simulink model "takeoff23b"  (R2025b)
settings: Solver=ode4  StartTime=0.0  StopTime=150  FixedStep=0.001  RelTol=1e-3
values from neighbouring files (symbols this model uses):
  a0 = 340.294    [basedata.m]    (also in basedata.mat; landing_init.m; landing_plan.mat; landingplan.mat)
  b_ref = 2.0    (= 2)    [basedata.m]    (also in basedata.mat; landing_init.m; landing_plan.mat; landingplan.mat)
  c_gear = [0.8e4, 1.4e4, 1.4e4]    [basedata.m]    (also in basedata.mat = [8000 14000 14000]; landing_init.m; landing_plan.mat = [8000 14000 14000]; landingplan.mat = [8000 14000 14000])
  c_lat = [1.4e4, 2.2e4, 2.2e4]    [basedata.m]    (also in basedata.mat = [14000 22000 22000]; landing_init.m; landing_plan.mat = [14000 22000 22000]; landingplan.mat = [14000 22000 22000])
  c_ref = 0.9    [basedata.m]    (also in basedata.mat; landing_init.m; landing_plan.mat; landingplan.mat)
  c_roll = [0.020, 0.018, 0.018]    [basedata.m]    (also in basedata.mat = [0.02 0.018 0.018]; landing_init.m; landing_plan.mat = [0.02 0.018 0.018]; landingplan.mat = [0.02 0.018 0.018])
  CD0 = 0.045    [basedata.m]    (also in basedata.mat; canshujisuan.m; landing_init.m; landing_plan.mat)
  CL0 = 0.083    [basedata.m]    (also in basedata.mat; landing_init.m; landing_plan.mat; landing_trajectory.m)
  CLa = 3.80    (= 3.8)    [basedata.m]    (also in basedata.mat; canshujisuan.m = 2.5; landing_init.m; landing_plan.mat)
  Clb = -0.08    [basedata.m]    (also in basedata.mat; landing_init.m; landing_plan.mat; landingplan.mat)
  Clda = -0.20    (= -0.2)    [basedata.m]    (also in basedata.mat; landing_init.m; landing_plan.mat; landingplan.mat)
  CLde = 0.28    [basedata.m]    (also in basedata.mat; landing_init.m; landing_plan.mat; landingplan.mat)
  Clp = -0.70    (= -0.7)    [basedata.m]    (also in basedata.mat; landing_init.m; landing_plan.mat; landingplan.mat)
  CLq = 4.50    (= 4.5)    [basedata.m]    (also in basedata.mat; canshujisuan.m = 3; landing_init.m; landing_plan.mat)
  Clr = 0.08    [basedata.m]    (also in basedata.mat; landing_init.m; landing_plan.mat; landingplan.mat)
  Cm0 = 0.060    (= 0.06)    [basedata.m]    (also in basedata.mat; landing_init.m; landing_plan.mat; landingplan.mat)
  Cma = -0.80    (= -0.8)    [basedata.m]    (also in basedata.mat; landing_init.m; landing_plan.mat; landingplan.mat)
  Cmde = -0.90    (= -0.9)    [basedata.m]    (also in basedata.mat; landing_init.m; landing_plan.mat; landingplan.mat)
  Cmq = -18.0    (= -18)    [basedata.m]    (also in basedata.mat; landing_init.m; landing_plan.mat; landingplan.mat)
  Cnb = 0.25    [basedata.m]    (also in basedata.mat; landing_init.m; landing_plan.mat; landingplan.mat)
  Cndr = -0.15    [basedata.m]    (also in basedata.mat; landing_init.m; landing_plan.mat; landingplan.mat)
  Cnp = -0.04    [basedata.m]    (also in basedata.mat; landing_init.m; landing_plan.mat; landingplan.mat)
  Cnr = -0.45    [basedata.m]    (also in basedata.mat; landing_init.m; landing_plan.mat; landingplan.mat)
  CSb = -0.70    (= -0.7)    [basedata.m]    (also in basedata.mat; landing_init.m; landing_plan.mat; landingplan.mat)
  CSdr = 0.18    [basedata.m]    (also in basedata.mat; landing_init.m; landing_plan.mat; landingplan.mat)
  CSr = 0.12    [basedata.m]    (also in basedata.mat; landing_init.m; landing_plan.mat; landingplan.mat)
  D = 0.5 * rho0 * V^2 * S_ref * CD_current    [canshujisuan.m]
  D0 = 1400    [basedata.m]    (also in basedata.mat; landing.m; landing_init.m; landing_plan.mat)
  da_max = 25    [basedata.m]    (also in basedata.mat; landing_init.m; landing_plan.mat; landingplan.mat)
  da_min = -da_max    (= -25)    [basedata.m]    (also in basedata.mat; landing_init.m; landing_plan.mat; landingplan.mat)
  de_max = 25    [basedata.m]    (also in basedata.mat; landing_init.m; landing_plan.mat; landingplan.mat)
  de_min = -de_max    (= -25)    [basedata.m]    (also in basedata.mat; landing_init.m; landing_plan.mat; landingplan.mat)
  DH = pi / 180    (= 0.0174532925199)    [basedata.m]    (also in basedata.mat; landing_init.m; landing_plan.mat; landingplan.mat)
  dr_max = 25    [basedata.m]    (also in basedata.mat; landing_init.m; landing_plan.mat; landingplan.mat)
  dr_min = -dr_max    (= -25)    [basedata.m]    (also in basedata.mat; landing_init.m; landing_plan.mat; landingplan.mat)
  g = 9.80665    [basedata.m]    (also in basedata.mat; canshujisuan.m; landing_init.m; landing_plan.mat)
  gamma1 = -0.125844364415    [basedata.mat]    (also in landing_trajectory.m = asin((T_idle - D_app) / (m*g)); landingplan.mat)
  gamma2 = -0.0261780104712    [basedata.mat]    (also in landing_trajectory.m; landingplan.mat)
  ground_z = 0.0    (= 0)    [basedata.m]    (also in basedata.mat; landing_init.m; landing_plan.mat; landingplan.mat)
  HD = 180 / pi    (= 57.2957795131)    [basedata.m]    (also in basedata.mat; landing_init.m; landing_plan.mat; landingplan.mat)
  I = [ Ixx, -Ixy, -Ixz ... (first row only)    [basedata.m]    (also in basedata.mat = [120  0  0; 0  480  0; 0  0  520]; landing_init.m; landing_plan.mat = [120  0  0; 0  480  0; 0  0  520]; landingplan.mat = [120  0  0; 0  480  0; 0  0  520])
  K = 0.12    [basedata.m]    (also in basedata.mat; canshujisuan.m = 0.08; landing_init.m; landing_plan.mat)
  K_alpha = 7.5375    [basedata.mat]    (also in control_design.m = (((wd_pitch^2)-a24))/(2*kesi_pitch*wd_pitch); control_design.mat; controller.m = 5; landingplan.mat)
  k_gear = [1.0e5, 3.0e5, 3.0e5]    [basedata.m]    (also in basedata.mat = [100000 300000 300000]; landing_init.m; landing_plan.mat = [100000 300000 300000]; landingplan.mat = [100000 300000 300000])
  Kn_pitch = -0.120095403309    [basedata.mat]    (also in control_design.m = -(2.2*g*(wd_pitch)^2)/(Tr*(((wd_pitch)^2)-a24)*V_control*a34; control_design.mat; controller.m = (2.2*wd^2*g)/(Tr*(wd^2-a24)*V_test*a34); landingplan.mat)
  Kw_pitch = -0.483749055178    [basedata.mat]    (also in control_design.m = -2*kesi_pitch*wd_pitch/a25; control_design.mat; controller.m = -(2*zeta*wd) / a25; landingplan.mat)
  m = 600.0    (= 600)    [basedata.m]    (also in basedata.mat; canshujisuan.m; landing_init.m; landing_plan.mat)
  mu_brake = [0.0, 0.55, 0.55]    [basedata.m]    (also in basedata.mat = [0 0.55 0.55]; landing_init.m; landing_plan.mat = [0 0.55 0.55]; landingplan.mat = [0 0.55 0.55])
  phi0 = 0.0    (= 0)    [landing.m]    (also in landing_init.m; landing_init.mat; landing_plan.mat; landingplan.mat)
  psi0 = 0.0    (= 0)    [landing.m]    (also in landing_init.m; landing_init.mat; landing_plan.mat; landingplan.mat)
  r_left_b = r_gear_b(:,2)    [basedata.m]    (also in basedata.mat = [-0.333333333333 -0.8 0.65]; landing_init.m; landing_plan.mat = [-0.333333333333 -0.8 0.65]; landingplan.mat = [-0.333333333333 -0.8 0.65])
  r_nose_b = r_gear_b(:,1)    [basedata.m]    (also in basedata.mat = [2 0 0.65]; landing_init.m; landing_plan.mat = [2 0 0.65]; landingplan.mat = [2 0 0.65])
  r_right_b = r_gear_b(:,3)    [basedata.m]    (also in basedata.mat = [-0.333333333333 0.8 0.65]; landing_init.m; landing_plan.mat = [-0.333333333333 0.8 0.65]; landingplan.mat = [-0.333333333333 0.8 0.65])
  rho0 = 1.225    [basedata.m]    (also in basedata.mat; canshujisuan.m; landing_init.m; landing_plan.mat)
  S_ref = 1.2    [basedata.m]    (also in basedata.mat; canshujisuan.m; landing_init.m; landing_plan.mat)
  theta0 = 0.0    (= 0)    [landing.m]    (also in landing_init.m; landing_init.mat = 0.0523598775598; landing_plan.mat = 0.0523560209424; landingplan.mat)
  u0_b = 128.0    (= 128)    [landing.m]    (also in landing_init.m; landing_init.mat = 100; landing_plan.mat; landingplan.mat)
  v0_b = 0.0    (= 0)    [landing.m]    (also in landing_init.m; landing_init.mat; landing_plan.mat; landingplan.mat)
  v_eps = 0.20    (= 0.2)    [basedata.m]    (also in basedata.mat; landing_init.m; landing_plan.mat; landingplan.mat)
  V_min = 3    [landing.m]    (also in landing_init.m; landing_plan.mat; landingplan.mat; plan.m = 1)
  w0_b = 0.0    (= 0)    [landing.m]    (also in landing_init.m; landing_init.mat; landing_plan.mat; landingplan.mat)
  wheel_radius = 0.18    [basedata.m]    (also in basedata.mat; landing_init.m; landing_plan.mat; landingplan.mat)
  WOW_on = 0.000    (= 0)    [basedata.m]    (also in basedata.mat; landing_init.m; landing_plan.mat; landingplan.mat)
  Xg0 = -12000.0    (= -12000)    [landing.m]    (also in landing_init.m; landing_init.mat = -8000; landing_plan.mat; landingplan.mat)
  Yg0 = 0.0    (= 0)    [landing.m]    (also in landing_init.m; landing_init.mat; landing_plan.mat; landingplan.mat)
  Zg0 = ground_z - wheel_radius - r_gear_b(3,1) + static_deflection    [basedata.m]    (also in basedata.mat = -0.8215943; landing.m = -1000; landing_init.m = -1000; landing_init.mat = -350)
undefined symbols (not defined in the file or in its folder): I_xz, I_yz, Ix_Iy, Iy_Iz, Iz_Ix
libraries: simulink x58, matrix_library x19
(part 2 of 4)

== system takeoff23b/Guidance/4_拉平制导 ==
  h_ALG : Inport
  h_dot : Inport  Port=2
  e_Z : Inport  Port=3
  e_psi : Inport  Port=4
  Enable : EnablePort
  Add : Sum  Inputs=+-
  Add1 : Sum  Inputs=+-
  Add2 : Sum
  Add3 : Sum  Inputs=+-
  Bus Creator : BusCreator  Inputs=10
  Constant : Constant  Value=-0.5
  Constant1 : Constant
  Constant2 : Constant  Value=0
  Constant3 : Constant  Value=0
  Gain : Gain  Gain=-1/2
  Gain1 : Gain  Gain=0.2
  Gain2 : Gain  Gain=-1
  Gain3 : Gain  Gain=-1
  Gain4 : Gain  Gain=0.02
  Gain5 : Gain  Gain=0.5
  H_cmd : Constant  Value=0
  Saturation : Saturate  UpperLimit=1.5  LowerLimit=0
  Saturation1 : Saturate  UpperLimit=0.17  LowerLimit=-0.17
  V_cmd : Constant  Value=200
  brake_cmd : Constant  Value=0
  gamma : Constant  Value=0
  theta_cmd : Constant  Value=0
  throttle_cmd : Constant  Value=0
  cmd_Bus : Outport
  wires:
  brake_cmd/1 -> Bus Creator/8  "brake_cmd"
  Saturation1/1 -> Bus Creator/4  "psi_cmd"
  V_cmd/1 -> Bus Creator/6  "V_cmd"
  throttle_cmd/1 -> Bus Creator/7  "throttle_cmd"
  Saturation/1 -> Bus Creator/1  "nz_cmd"
  theta_cmd/1 -> Bus Creator/5  "theta_cmd"
  Constant3/1 -> Bus Creator/2  "ny_cmd"
  Bus Creator/1 -> cmd_Bus/1
  Constant2/1 -> Bus Creator/3  "phi_cmd"
  h_ALG/1 -> Add/1
  Constant/1 -> Add/2
  Add/1 -> Gain/1
  h_dot/1 -> Add1/1
  Gain/1 -> Add1/2
  Gain1/1 -> Add2/1
  Add1/1 -> Gain1/1
  Constant1/1 -> Add2/2
  Add2/1 -> Saturation/1
  e_Z/1 -> Gain2/1
  e_psi/1 -> Gain3/1
  Gain2/1 -> Gain4/1
  Gain3/1 -> Gain5/1
  Gain4/1 -> Add3/1
  Gain5/1 -> Add3/2
  Add3/1 -> Saturation1/1
  H_cmd/1 -> Bus Creator/10  "H_cmd"
  gamma/1 -> Bus Creator/9  "gamma"

== system takeoff23b/controller1/1_Pitch_Ctrl ==
  Flight_Phase : Inport
  nz_cmd : Inport  Port=2
  theta_cmd : Inport  Port=3
  nz : Inport  Port=4
  theta : Inport  Port=5
  q : Inport  Port=6
  H_cmd : Inport  Port=7
  gamma : Inport  Port=8
  234俯仰角控制 : Subsystem
  5_着陆俯仰控制 : Subsystem
  5三回路控制 : Subsystem
  Clock_blend : Clock
  Compare To Constant1 : simulink/Logic and Bit Operations/Compare To Constant  relop=>=  const=6  OutDataTypeStr=boolean
  Compare To Constant2 : simulink/Logic and Bit Operations/Compare To Constant  relop=>=  const=5  OutDataTypeStr=boolean
  Compare To Constant3 : simulink/Logic and Bit Operations/Compare To Constant  relop=<=  const=9  OutDataTypeStr=boolean
  Compare To Constant4 : simulink/Logic and Bit Operations/Compare To Constant  relop=<=  const=7  OutDataTypeStr=boolean
  Gain3 : Gain  Gain=180/pi
  Logical Operator1 : Logic  AllPortsSameDT=off  OutDataTypeStr=boolean
  Logical Operator2 : Logic  Operator=NOT  AllPortsSameDT=off  OutDataTypeStr=boolean
  Logical Operator3 : Logic  AllPortsSameDT=off  OutDataTypeStr=boolean
  Pitch45Blend : MATLAB Function  TreatAsAtomicUnit=on  SystemSampleTime=0.001
  Saturation : Saturate  UpperLimit=25  LowerLimit=-25
  Scope1 : Scope
      settings: ActiveDisplayYMinimum=-0.125  ActiveDisplayYMaximum=1.125
  Scope2 : Scope
      settings: ActiveDisplayYMinimum=-3.5044630346224475  ActiveDisplayYMaximum=0.72101097537351044  DataLoggingVariableName=ScopeData30
  Switch : Switch  Criteria=u2 > Threshold  SaturateOnIntegerOverflow=off  InputSameDT=off
  T_blend : Constant  Value=5
  de_cmd : Outport
  wires:
  Pitch45Blend/1(de_cmd_rad) -> Gain3/1
  Compare To Constant3/1 -> Logical Operator1/1
  Compare To Constant2/1 -> Logical Operator1/2
  Logical Operator1/1 -> Logical Operator2/1
  Flight_Phase/1 -> Compare To Constant3/1, Pitch45Blend/1(phase), Compare To Constant4/1, Compare To Constant1/1, Compare To Constant2/1
  Clock_blend/1 -> Pitch45Blend/4(t)
  Pitch45Blend/2(lambda) -> Scope1/1
  T_blend/1 -> Pitch45Blend/5(T_blend)
  Gain3/1 -> Saturation/1
  theta_cmd/1 -> 234俯仰角控制/1(theta_cmd)
  theta/1 -> 234俯仰角控制/2(theta)
  nz_cmd/1 -> 5三回路控制/1(nz_cmd)
  nz/1 -> 5三回路控制/2(nz)
  q/1 -> 234俯仰角控制/3(q), 5三回路控制/3(q)
  Logical Operator2/1 -> 5三回路控制/4(复位)
  234俯仰角控制/1(de_theta_rad) -> Pitch45Blend/2(de_theta_rad)
  5三回路控制/1(de_nz_rad) -> Switch/1, Pitch45Blend/3(de_ny_rad)
  Compare To Constant1/1 -> Logical Operator3/2
  Compare To Constant4/1 -> Logical Operator3/1
  Logical Operator3/1 -> Switch/2
  Switch/1 -> Scope2/1, de_cmd/1
  5_着陆俯仰控制/1(de) -> Switch/3
  [Vg] -> 5_着陆俯仰控制/1(Vg)
  H_cmd/1 -> 5_着陆俯仰控制/3(h_com)
  gamma/1 -> 5_着陆俯仰控制/2(gamma)

== system takeoff23b/controller1/2_Yaw_Ctrl ==
  Flight_Phase : Inport
  psi_cmd : Inport  Port=2
  Y : Inport  Port=3
  psi : Inport  Port=4
  r : Inport  Port=5
  2345上升段控制 : Subsystem
  Compare To Constant : simulink/Logic and Bit Operations/Compare To Constant  relop=>=  const=1  OutDataTypeStr=boolean
  Compare To Constant1 : simulink/Logic and Bit Operations/Compare To Constant  relop=<=  const=8  OutDataTypeStr=boolean
  Compare To Constant2 : simulink/Logic and Bit Operations/Compare To Constant  relop===  const=1  OutDataTypeStr=boolean
  Compare To Constant3 : simulink/Logic and Bit Operations/Compare To Constant  relop===  const=10  OutDataTypeStr=boolean
  Compare To Constant4 : simulink/Logic and Bit Operations/Compare To Constant  relop===  const=11  OutDataTypeStr=boolean
  Constant : Constant  Value=0
  Constant1 : Constant  Value=0
  Gain : Gain  Gain=180/pi
  Gain1 : Gain  Gain=180/pi
  Logical Operator : Logic  AllPortsSameDT=off  OutDataTypeStr=boolean
  Logical Operator1 : Logic  Operator=OR  Inputs=3  AllPortsSameDT=off  OutDataTypeStr=boolean
  Saturation : Saturate  UpperLimit=25  LowerLimit=-25
  Saturation1 : Saturate  UpperLimit=25  LowerLimit=-25
  Scope : Scope
      settings: ActiveDisplayYMinimum=-0.036  ActiveDisplayYMaximum=0.004
  Switch : Switch  Criteria=u2 > Threshold  SaturateOnIntegerOverflow=off  InputSameDT=off
  Switch1 : Switch  Criteria=u2 > Threshold  SaturateOnIntegerOverflow=off  InputSameDT=off
  dr_cmd : Outport
  delta_s_cmd : Outport  Port=2
  wires:
  Gain/1 -> Saturation/1
  Saturation/1 -> dr_cmd/1
  Saturation1/1 -> delta_s_cmd/1
  Gain1/1 -> Saturation1/1
  Compare To Constant/1 -> Logical Operator/1
  Compare To Constant1/1 -> Logical Operator/2
  Logical Operator/1 -> Switch/2
  Compare To Constant3/1 -> Logical Operator1/2
  Compare To Constant2/1 -> Logical Operator1/1
  Compare To Constant4/1 -> Logical Operator1/3
  Logical Operator1/1 -> Switch1/2
  Constant/1 -> Switch1/3
  Flight_Phase/1 -> Compare To Constant/1, Compare To Constant1/1, Compare To Constant2/1, Compare To Constant3/1, Compare To Constant4/1
  Constant1/1 -> Switch/3  "阶段9"
  Switch1/1 -> Gain1/1
  Switch/1 -> Gain/1
  2345上升段控制/1(dr_cmd) -> Switch/1
  psi_cmd/1 -> Switch1/1
  Y/1 -> 2345上升段控制/1(Y)
  psi/1 -> Scope/1, 2345上升段控制/2(psi)
  r/1 -> 2345上升段控制/3(r)
  [Vwind_ground] -> 2345上升段控制/4(Vwind_ground)
  [Va_safe] -> 2345上升段控制/5(Va_safe)

== system takeoff23b/controller1/3_Roll_Ctrl ==
  phi_cmd : Inport
  phi : Inport  Port=2
  p : Inport  Port=3
  Gain : Gain  Gain=180/pi
  Gain1 : Gain
  Gain2 : Gain  Gain=5
  Gain3 : Gain  Gain=0.1
  Gain4 : Gain  Gain=-1
  Integrator : Integrator
  Saturation : Saturate  UpperLimit=25  LowerLimit=-25
  Saturation1 : Saturate  UpperLimit=0.52  LowerLimit=-0.52
  Sum : Sum  Inputs=|+-
  Sum1 : Sum  Inputs=|++
  Sum2 : Sum  Inputs=|+-
  da_cmd : Outport
  wires:
  Gain/1 -> Saturation/1
  Saturation/1 -> Gain4/1
  phi_cmd/1 -> Sum/1
  phi/1 -> Sum/2
  Sum/1 -> Saturation1/1
  Gain3/1 -> Integrator/1
  Integrator/1 -> Sum1/2
  Gain2/1 -> Sum1/1
  Sum1/1 -> Sum2/1
  p/1 -> Sum2/2
  Sum2/1 -> Gain1/1
  Saturation1/1 -> Gain2/1, Gain3/1
  Gain1/1 -> Gain/1
  Gain4/1 -> da_cmd/1

== system takeoff23b/controller1/4_Power&V_Ctrl ==
  Flight_Phase : Inport
  V_cmd : Inport  Port=2
  throttle_cmd : Inport  Port=3
  V : Inport  Port=4
  brake_cmd : Inport  Port=5
  Clock_blend : Clock
  Constant : Constant  Value=3
  Delay : Delay  DelayLength=1
  Gain : Gain  Gain=0.1
  Gain1 : Gain  Gain=0.08
  MATLAB Function : MATLAB Function  TreatAsAtomicUnit=on
  MATLAB Function1 : MATLAB Function  TreatAsAtomicUnit=on
  Max : MinMax  Function=max  Inputs=2
  Saturation : Saturate  UpperLimit=0.55  LowerLimit=-0.45
  Saturation1 : Saturate  UpperLimit=1  LowerLimit=0
  Saturation2 : Saturate  UpperLimit=1  LowerLimit=0
  Scope : Scope
      settings: DataLoggingVariableName=ScopeData3
  Sum1 : Sum  Inputs=|+-
  Sum2 : Sum  Inputs=|++
  Sum3 : Sum  Inputs=|+-
  平衡油门 : Constant  Value=0.45
  最小爬升油门保护 : Constant  Value=0.3
  throttle : Outport
  u_brake_cmd : Outport  Port=2
  wires:
  Saturation1/1 -> u_brake_cmd/1
  V/1 -> Sum3/2
  V_cmd/1 -> Sum3/1
  brake_cmd/1 -> Saturation1/1
  Sum3/1 -> Gain/1
  Gain/1 -> Sum1/1
  Sum1/1 -> Saturation/1
  平衡油门/1 -> Sum2/2
  [vg_xyz] -> MATLAB Function/1(Vel_g)
  [a_xyz] -> MATLAB Function/2(axyz)
  MATLAB Function/1(dv_err) -> Delay/1
  Gain1/1 -> Sum1/2
  Saturation/1 -> Sum2/1
  Sum2/1 -> Max/1
  Clock_blend/1 -> MATLAB Function1/4(t)
  throttle_cmd/1 -> MATLAB Function1/2(throttle_direct)
  Max/1 -> MATLAB Function1/3(throttle_speed)
  Flight_Phase/1 -> MATLAB Function1/1(phase)
  Constant/1 -> MATLAB Function1/5(T_blend)
  MATLAB Function1/1(throttle_out) -> Saturation2/1
  MATLAB Function1/2(lambda) -> Scope/1
  Delay/1 -> Gain1/1
  Saturation2/1 -> throttle/1

== system takeoff23b/controller1/刹车 ==
  u_brake_cmd : Inport
  Gain : Gain  Gain=1/0.1
  Integrator : Integrator  LimitOutput=on  UpperSaturationLimit=1  LowerSaturationLimit=0
  Sum : Sum  Inputs=|+-
  限制舵面角速度 : Saturate  UpperLimit=5  LowerLimit=-5
  u_brake : Outport
  wires:
  u_brake_cmd/1 -> Sum/1
  Sum/1 -> Gain/1
  Gain/1 -> 限制舵面角速度/1
  限制舵面角速度/1 -> Integrator/1
  Integrator/1 -> Sum/2, u_brake/1

== system takeoff23b/controller1/前轮 ==
  delta_s_cmd : Inport
  Gain : Gain  Gain=1/0.08
  Integrator : Integrator  LimitOutput=on  UpperSaturationLimit=25  LowerSaturationLimit=-25
  Sum : Sum  Inputs=|+-
  限制偏转速度 : Saturate  UpperLimit=120  LowerLimit=-120
  delta_s : Outport
  wires:
  delta_s_cmd/1 -> Sum/1
  Sum/1 -> Gain/1
  Gain/1 -> 限制偏转速度/1
  限制偏转速度/1 -> Integrator/1
  Integrator/1 -> Sum/2, delta_s/1

== system takeoff23b/controller1/副翼 ==
  da_cmd : Inport
  Gain : Gain  Gain=1/0.05
  Integrator : Integrator  LimitOutput=on  UpperSaturationLimit=25  LowerSaturationLimit=-25
  Sum : Sum  Inputs=|+-
  限制舵面角速度 : Saturate  UpperLimit=120  LowerLimit=-120
  da : Outport
  wires:
  da_cmd/1 -> Sum/1
  Sum/1 -> Gain/1
  Gain/1 -> 限制舵面角速度/1
  限制舵面角速度/1 -> Integrator/1
  Integrator/1 -> Sum/2, da/1

== system takeoff23b/controller1/升降舵 ==
  de_cmd : Inport
  Gain : Gain  Gain=1/0.08
  Integrator : Integrator  LimitOutput=on  UpperSaturationLimit=25  LowerSaturationLimit=-25
  Sum : Sum  Inputs=|+-
  限制舵面角速度 : Saturate  UpperLimit=50  LowerLimit=-50
  de : Outport
  wires:
  de_cmd/1 -> Sum/1
  Sum/1 -> Gain/1
  Gain/1 -> 限制舵面角速度/1
  限制舵面角速度/1 -> Integrator/1
  Integrator/1 -> Sum/2, de/1

== system takeoff23b/controller1/方向舵 ==
  dr_cmd : Inport
  Gain : Gain  Gain=1/0.05
  Integrator : Integrator  LimitOutput=on  UpperSaturationLimit=25  LowerSaturationLimit=-25
  Sum : Sum  Inputs=|+-
  限制舵面角速度 : Saturate  UpperLimit=100  LowerLimit=-100
  dr : Outport
  wires:
  Integrator/1 -> dr/1, Sum/2
  限制舵面角速度/1 -> Integrator/1
  Gain/1 -> 限制舵面角速度/1
  Sum/1 -> Gain/1
  dr_cmd/1 -> Sum/1

== system takeoff23b/controller1/油门 ==
  throttle : Inport
  Constant : Constant  Value=3000
  Gain : Gain  Gain=1/0.5
  Integrator : Integrator  LimitOutput=on  UpperSaturationLimit=1  LowerSaturationLimit=0
  Product : Product
  Saturation : Saturate  UpperLimit=3  LowerLimit=-3
  Sum : Sum  Inputs=|+-
  thrust : Outport
  wires:
  Integrator/1 -> Product/2, Sum/2
  Saturation/1 -> Integrator/1
  Gain/1 -> Saturation/1
  Sum/1 -> Gain/1
  throttle/1 -> Sum/1
  Product/1 -> thrust/1
  Constant/1 -> Product/1

== system takeoff23b/6DOF-MODEL/AERO-PARAMETER/atmosphere ==
  Constant : Constant  Value=0
  Constant1 : Constant  Value=rho0
  Constant2 : Constant  Value=a0
  Constant3 : Constant  Value=0.5
  Constant4 : Constant  Value=0
  Constant5 : Constant  Value=0
  Display : Display
  MATLAB Function : MATLAB Function  TreatAsAtomicUnit=on
  Matrix Multiply : Product  Multiplication=Matrix(*)
  Mux : Mux  Inputs=3
  Product : Product  Inputs=3
  Reshape : Reshape  OutputDimensionality=Column vector (2-D)
  Square : Math  Operator=square
  tag scope: Vwind_body=global, Vwind_ground=global, a_sound=global, qc=global, rho=global
  wires:
  Constant1/1 -> [rho]
  Constant2/1 -> [a_sound]
  Constant3/1 -> Product/1
  [rho] -> Product/2
  Product/1 -> Display/1, [qc]
  Square/1 -> Product/3
  [Vg] -> Square/1
  Constant5/1 -> Mux/2
  Constant4/1 -> Mux/1
  Constant/1 -> Mux/3
  Mux/1 -> Reshape/1
  Reshape/1 -> [Vwind_ground]
  [Vwind_ground] -> Matrix Multiply/2
  [theta_eular] -> MATLAB Function/2(theta)
  [phi_eular] -> MATLAB Function/1(phi)
  MATLAB Function/1(R_bg) -> Matrix Multiply/1
  [psi_eular] -> MATLAB Function/3(psi)
  Matrix Multiply/1 -> [Vwind_body]

== system takeoff23b/6DOF-MODEL/AERO-PARAMETER/侧向力系数 ==
  beta(H) : Inport
  dr(H) : Inport  Port=2
  Add : Sum  Inputs=+++
  Constant1 : Constant  Value=CSb
  Constant2 : Constant  Value=CSr
  Constant3 : Constant  Value=CSdr
  Product : Product
  Product2 : Product
  Product3 : Product
  CS : Outport
  wires:
  Add/1 -> CS/1
  Constant3/1 -> Product2/2
  Product2/1 -> Add/3
  dr(H)/1 -> Product2/1
  beta(H)/1 -> Product/1
  Constant1/1 -> Product/2
  Constant2/1 -> Product3/2
  [r_hat] -> Product3/1
  Product/1 -> Add/1
  Product3/1 -> Add/2

== system takeoff23b/6DOF-MODEL/AERO-PARAMETER/俯仰力矩系数 ==
  alpha(H) : Inport
  de(H) : Inport  Port=2
  Add : Sum  Inputs=++++
  Constant : Constant  Value=Cm0
  Constant1 : Constant  Value=Cma
  Constant2 : Constant  Value=Cmq
  Constant3 : Constant  Value=Cmde
  Product : Product
  Product2 : Product
  Product3 : Product
  Cm : Outport
  wires:
  Product2/1 -> Add/4
  de(H)/1 -> Product2/1
  Constant3/1 -> Product2/2
  alpha(H)/1 -> Product/1
  Constant1/1 -> Product/2
  Add/1 -> Cm/1
  Constant2/1 -> Product3/2
  [q_hat] -> Product3/1
  Product3/1 -> Add/3
  Product/1 -> Add/2
  Constant/1 -> Add/1

== system takeoff23b/6DOF-MODEL/AERO-PARAMETER/偏航力矩系数 ==
  beta(H) : Inport
  dr(H) : Inport  Port=2
  Add : Sum  Inputs=++++
  Constant1 : Constant  Value=Cnb
  Constant2 : Constant  Value=Cnp
  Constant3 : Constant  Value=Cndr
  Constant4 : Constant  Value=Cnr
  Product{,1..3} (4 alike) : Product
  Cn : Outport
  wires:
  Product2/1 -> Add/4
  Constant4/1 -> Product1/2
  Product/1 -> Add/1
  dr(H)/1 -> Product2/1
  Constant3/1 -> Product2/2
  beta(H)/1 -> Product/1
  Constant1/1 -> Product/2
  Add/1 -> Cn/1
  Constant2/1 -> Product3/2
  [p_hat] -> Product3/1
  Product1/1 -> Add/3
  [r_hat] -> Product1/1
  Product3/1 -> Add/2

== system takeoff23b/6DOF-MODEL/AERO-PARAMETER/力矩系数2力矩 ==
  Cl/Cm/Cn : Inport
  Constant : Constant  Value=S_ref
  Constant1 : Constant  Value=c_ref
  Constant2 : Constant  Value=b_ref
  Demux : Demux  Outputs=3
  Mux : Mux  Inputs=3
  Product : Product  Inputs=4
  Product1 : Product  Inputs=4
  Product2 : Product  Inputs=4
  MX/MY/MZ : Outport
  wires:
  Cl/Cm/Cn/1 -> Demux/1
  Demux/1 -> Product/1
  Constant/1 -> Product/2, Product1/2, Product2/2
  Demux/3 -> Product2/1
  Demux/2 -> Product1/1
  [qc] -> Product/3, Product2/3, Product1/3
  Product/1 -> Mux/1
  Product1/1 -> Mux/2
  Product2/1 -> Mux/3
  Mux/1 -> MX/MY/MZ/1
  Constant2/1 -> Product/4, Product2/4
  Constant1/1 -> Product1/4

== system takeoff23b/6DOF-MODEL/AERO-PARAMETER/力系数2力 ==
  CD/CL/CS : Inport
  Constant : Constant  Value=S_ref
  Demux : Demux  Outputs=3
  Display : Display
  Display1 : Display
  Display2 : Display
  Gain : Gain  Gain=-1
  Gain1 : Gain  Gain=-1
  Mux : Mux  Inputs=3
  Product : Product  Inputs=3
  Product1 : Product  Inputs=3
  Product2 : Product  Inputs=3
  D/L/S : Outport
  wires:
  CD/CL/CS/1 -> Demux/1
  Demux/1 -> Product/1
  Constant/1 -> Product2/2, Product1/2, Product/2
  Demux/3 -> Product2/1
  Demux/2 -> Product1/1
  [qc] -> Product2/3, Product1/3, Product/3
  Product/1 -> Display/1, Gain/1
  Product1/1 -> Display1/1, Gain1/1
  Product2/1 -> Display2/1, Mux/3
  Mux/1 -> D/L/S/1
  Gain/1 -> Mux/1
  Gain1/1 -> Mux/2

== system takeoff23b/6DOF-MODEL/AERO-PARAMETER/升力系数 ==
  alpha(H) : Inport
  de(H) : Inport  Port=2
  Add : Sum  Inputs=++++
  Constant : Constant  Value=CL0
  Constant1 : Constant  Value=CLa
  Constant2 : Constant  Value=CLq
  Constant3 : Constant  Value=CLde
  Product : Product
  Product2 : Product
  Product3 : Product
  CL : Outport
  wires:
  Constant/1 -> Add/1
  alpha(H)/1 -> Product/1
  Constant1/1 -> Product/2
  Product/1 -> Add/2
  [q_hat] -> Product3/1
  Constant2/1 -> Product3/2
  de(H)/1 -> Product2/1
  Constant3/1 -> Product2/2
  Product2/1 -> Add/4
  Product3/1 -> Add/3
  Add/1 -> CL/1

== system takeoff23b/6DOF-MODEL/AERO-PARAMETER/无量纲化角速率 ==
  p : Inport
  q : Inport  Port=2
  r : Inport  Port=3
  Constant : Constant  Value=V_min
  Max : MinMax  Function=max  Inputs=2
  Scope : Scope
      settings: ActiveDisplayYMinimum=-0.00063  ActiveDisplayYMaximum=7E-5  DataLoggingVariableName=ScopeData21
  Subsystem : Subsystem
  Subsystem1 : Subsystem
  Subsystem2 : Subsystem
  tag scope: Va_safe=global, p_hat=global, q_hat=global, r_hat=global
  wires:
  p/1 -> Subsystem2/1(p)
  [Va_safe] -> Subsystem2/2(Va), Subsystem1/2(Va), Subsystem/2(Va)
  Subsystem/1(r_hat) -> [r_hat]
  Subsystem1/1(q_hat) -> Scope/1, [q_hat]
  Subsystem2/1(p_hat) -> [p_hat]
  [Va] -> Max/2
  Constant/1 -> Max/1
  Max/1 -> [Va_safe]
  r/1 -> Subsystem/1(r)
  q/1 -> Subsystem1/1(q)

== system takeoff23b/6DOF-MODEL/AERO-PARAMETER/滚转力矩系数 ==
  beta(H) : Inport
  da(H) : Inport  Port=2
  Add : Sum  Inputs=++++
  Constant1 : Constant  Value=Clb
  Constant2 : Constant  Value=Clp
  Constant3 : Constant  Value=Clda
  Constant4 : Constant  Value=Clr
  Product{,1..3} (4 alike) : Product
  Cl : Outport
  wires:
  Product3/1 -> Add/2
  da(H)/1 -> Product2/1
  Product/1 -> Add/1
  beta(H)/1 -> Product/1
  Add/1 -> Cl/1
  Constant1/1 -> Product/2
  Constant3/1 -> Product2/2
  Constant2/1 -> Product3/2
  [p_hat] -> Product3/1
  Product1/1 -> Add/3
  [r_hat] -> Product1/1
  Constant4/1 -> Product1/2
  Product2/1 -> Add/4

== system takeoff23b/6DOF-MODEL/AERO-PARAMETER/阻力系数 ==
  Add : Sum
  Constant : Constant  Value=CD0
  Constant1 : Constant  Value=K
  Product : Product
  Square : Math  Operator=square
  CD : Outport
  wires:
  Constant/1 -> Add/1
  Constant1/1 -> Product/1
  [CL] -> Square/1
  Square/1 -> Product/2
  Product/1 -> Add/2
  Add/1 -> CD/1

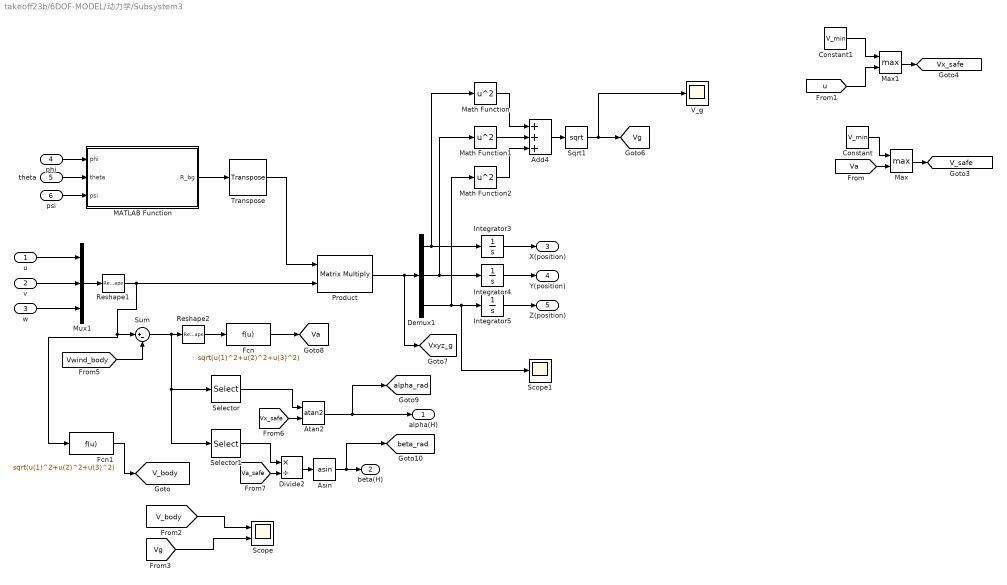
== system takeoff23b/6DOF-MODEL/动力学/Subsystem3 ==
  u : Inport
  v : Inport  Port=2
  w : Inport  Port=3
  phi : Inport  Port=4
  theta : Inport  Port=5
  psi : Inport  Port=6
  Add4 : Sum  Inputs=+++
  Asin : Trigonometry  Operator=asin
  Atan2 : Trigonometry  Operator=atan2
  Constant : Constant  Value=V_min
  Constant1 : Constant  Value=V_min  VectorParams1D=off
  Demux1 : Demux  Outputs=3
  Divide2 : Product  Inputs=*/
  Fcn : Fcn  Expr=sqrt(u(1)^2+u(2)^2+u(3)^2)
  Fcn1 : Fcn  Expr=sqrt(u(1)^2+u(2)^2+u(3)^2)
  Integrator3 : Integrator  InitialCondition=Xg0
  Integrator4 : Integrator  InitialCondition=Yg0
  Integrator5 : Integrator  InitialCondition=Zg0
  MATLAB Function : MATLAB Function  TreatAsAtomicUnit=on
  Math Function : Math  Operator=square
  Math Function1 : Math  Operator=square
  Math Function2 : Math  Operator=square
  Max : MinMax  Function=max  Inputs=2
  Max1 : MinMax  Function=max  Inputs=2
  Mux1 : Mux  Inputs=3
  Product : Product  Multiplication=Matrix(*)
  Reshape1 : Reshape  OutputDimensionality=Column vector (2-D)
  Reshape2 : Reshape
  Scope : Scope  NumInputPorts=2
      settings: ActiveDisplayYMinimum=-33.7401  ActiveDisplayYMaximum=303.6609  DataLoggingVariableName=ScopeData3
  Scope1 : Scope
      settings: ActiveDisplayYMinimum=-1.7327376089193578  ActiveDisplayYMaximum=6.8260938777848246  DataLoggingVariableName=ScopeData31
  Selector : Selector  InputPortWidth=3  IndexOptions=Index vector (dialog)  Indices=3  OutputSizes=1
  Selector1 : Selector  InputPortWidth=3  IndexOptions=Index vector (dialog)  Indices=2  OutputSizes=1
  Sqrt1 : Sqrt
  Sum : Sum  Inputs=|+-
  Transpose : matrix_library/Transpose
  V_g : Scope
      settings: ActiveDisplayYMinimum=31.0917  ActiveDisplayYMaximum=62.5187
  alpha(H) : Outport
  beta(H) : Outport  Port=2
  X(position) : Outport  Port=3
  Y(position) : Outport  Port=4
  Z(position) : Outport  Port=5
  tag scope: V_body=global, V_safe=global, Va=global, Vg=global, Vx_safe=global, Vxyz_g=global, alpha_rad=global, beta_rad=global
  wires:
  Constant/1 -> Max/1
  Max/1 -> [V_safe]
  [Va] -> Max/2
  Constant1/1 -> Max1/1
  Max1/1 -> [Vx_safe]
  [u] -> Max1/2
  phi/1 -> MATLAB Function/1(phi)
  Demux1/2 -> Math Function1/1, Integrator4/1
  Demux1/1 -> Math Function/1, Integrator3/1
  Fcn/1 -> [Va]
  Product/1 -> [Vxyz_g], Demux1/1
  Mux1/1 -> Reshape1/1
  theta/1 -> MATLAB Function/2(theta)
  u/1 -> Mux1/1
  Math Function2/1 -> Add4/3
  Reshape2/1 -> Fcn/1
  v/1 -> Mux1/2
  Demux1/3 -> Math Function2/1, Scope1/1, Integrator5/1
  MATLAB Function/1(R_bg) -> Transpose/1
  Sum/1 -> Selector1/1, Selector/1, Reshape2/1
  Add4/1 -> Sqrt1/1
  Math Function/1 -> Add4/1
  Math Function1/1 -> Add4/2
  psi/1 -> MATLAB Function/3(psi)
  Atan2/1 -> [alpha_rad], alpha(H)/1
  Sqrt1/1 -> [Vg], V_g/1
  Reshape1/1 -> Fcn1/1, Sum/1, Product/2
  Transpose/1 -> Product/1
  w/1 -> Mux1/3
  Integrator3/1 -> X(position)/1
  Integrator4/1 -> Y(position)/1
  Integrator5/1 -> Z(position)/1
  [Vwind_body] -> Sum/2
  [Vx_safe] -> Atan2/2
  Selector/1 -> Atan2/1
  [Va_safe] -> Divide2/2
  Selector1/1 -> Divide2/1
  Divide2/1 -> Asin/1
  Asin/1 -> [beta_rad], beta(H)/1
  Fcn1/1 -> [V_body]
  [V_body] -> Scope/1
  [Vg] -> Scope/2

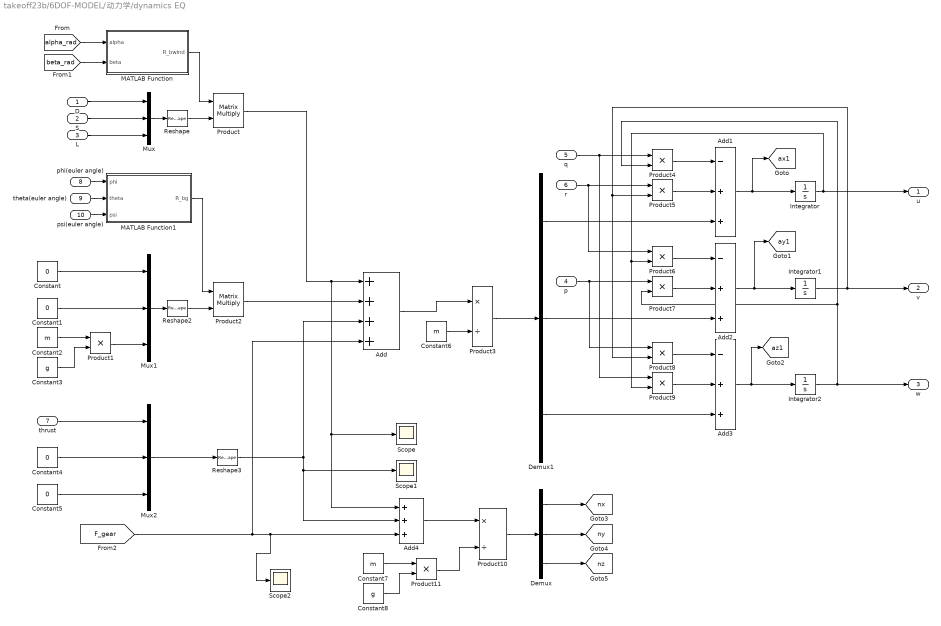
== system takeoff23b/6DOF-MODEL/动力学/dynamics EQ ==
  D : Inport
  S : Inport  Port=2
  L : Inport  Port=3
  p : Inport  Port=4
  q : Inport  Port=5
  r : Inport  Port=6
  thrust : Inport  Port=7
  phi(euler angle) : Inport  Port=8
  theta(euler angle) : Inport  Port=9
  psi(euler angle) : Inport  Port=10
  Add : Sum  Inputs=++++
  Add1 : Sum  Inputs=-++
  Add2 : Sum  Inputs=-++
  Add3 : Sum  Inputs=-++
  Add4 : Sum  Inputs=+++
  Constant{,1,4..5} (4 alike) : Constant  Value=0
  Constant2 : Constant  Value=m
  Constant3 : Constant  Value=g
  Constant6 : Constant  Value=m
  Constant7 : Constant  Value=m
  Constant8 : Constant  Value=g
  Demux : Demux  Outputs=3
  Demux1 : Demux  Outputs=3
  Integrator : Integrator  InitialCondition=u0_b
  Integrator1 : Integrator  InitialCondition=v0_b
  Integrator2 : Integrator  InitialCondition=w0_b
  MATLAB Function : MATLAB Function  TreatAsAtomicUnit=on
  MATLAB Function1 : MATLAB Function  TreatAsAtomicUnit=on
  Mux : Mux  Inputs=3
  Mux1 : Mux  Inputs=3
  Mux2 : Mux  Inputs=3
  Product : Product  Multiplication=Matrix(*)
  Product{1,4..9,11} (8 alike) : Product
  Product10 : Product  Inputs=*/
  Product2 : Product  Multiplication=Matrix(*)
  Product3 : Product  Inputs=*/
  Reshape : Reshape  OutputDimensionality=Column vector (2-D)
  Reshape2 : Reshape  OutputDimensionality=Column vector (2-D)
  Reshape3 : Reshape  OutputDimensionality=Column vector (2-D)
  Scope : Scope
      settings: ActiveDisplayYMinimum=-81.5338  ActiveDisplayYMaximum=28.5748  DataLoggingVariableName=ScopeData2
  Scope1 : Scope
      settings: ActiveDisplayYMinimum=-375  ActiveDisplayYMaximum=3375  DataLoggingVariableName=ScopeData3
  Scope2 : Scope
      settings: ActiveDisplayYMinimum=-5.497925726682791E+86  ActiveDisplayYMaximum=4.9481331540145126E+87  DataLoggingVariableName=ScopeData4
  u : Outport
  v : Outport  Port=2
  w : Outport  Port=3
  tag scope: ax1=global, ay1=global, az1=global, nx=global, ny=global, nz=global
  wires:
  S/1 -> Mux/2
  D/1 -> Mux/1
  L/1 -> Mux/3
  Mux/1 -> Reshape/1
  Reshape/1 -> Product/2
  MATLAB Function/1(R_bwind) -> Product/1
  thrust/1 -> Mux2/1
  theta(euler angle)/1 -> MATLAB Function1/2(theta)
  phi(euler angle)/1 -> MATLAB Function1/1(phi)
  psi(euler angle)/1 -> MATLAB Function1/3(psi)
  Constant2/1 -> Product1/1
  Constant3/1 -> Product1/2
  Constant1/1 -> Mux1/2
  Constant/1 -> Mux1/1
  Product1/1 -> Mux1/3
  Mux1/1 -> Reshape2/1
  Reshape2/1 -> Product2/2
  Constant4/1 -> Mux2/2
  Constant5/1 -> Mux2/3
  Mux2/1 -> Reshape3/1
  Add/1 -> Product3/1
  Product3/1 -> Demux1/1
  Add1/1 -> [ax1], Integrator/1
  MATLAB Function1/1(R_bg) -> Product2/1
  Product2/1 -> Add/2
  Reshape3/1 -> Add4/2, Scope1/1, Add/3
  Product/1 -> Add/1, Add4/1, Scope/1
  Constant6/1 -> Product3/2
  Demux1/1 -> Add1/3
  Product5/1 -> Add1/2
  r/1 -> Product6/1, Product5/1
  q/1 -> Product9/1, Product4/1
  Demux1/2 -> Add2/3
  Product7/1 -> Add2/2
  Product4/1 -> Add1/1
  Product6/1 -> Add2/1
  Product8/1 -> Add3/1
  Product9/1 -> Add3/2
  Demux1/3 -> Add3/3
  p/1 -> Product8/1, Product7/1
  Integrator/1 -> Product6/2, Product9/2, u/1
  Add2/1 -> [ay1], Integrator1/1
  Integrator1/1 -> Product8/2, Product5/2, v/1
  Add3/1 -> [az1], Integrator2/1
  Integrator2/1 -> Product7/2, Product4/2, w/1
  Add4/1 -> Product10/1
  Product11/1 -> Product10/2
  Constant8/1 -> Product11/2
  Constant7/1 -> Product11/1
  Product10/1 -> Demux/1
  Demux/1 -> [nx]
  Demux/2 -> [ny]
  Demux/3 -> [nz]
  [alpha_rad] -> MATLAB Function/1(alpha)
  [beta_rad] -> MATLAB Function/2(beta)
  [F_gear] -> Scope2/1, Add4/3, Add/4

== system takeoff23b/6DOF-MODEL/动力学/height ==
  Constant : Constant  Value=ground_z
  Constant1 : Constant  Commented=on  Value=0
  Constant2 : Constant  Commented=on
  Demux1 : Demux  Outputs=3
  Demux2 : Demux  Outputs=3
  From : From  Commented=on  GotoTag=height  TagVisibility=global
  Hermitian Transpose1 : matrix_library/Hermitian Transpose
  Hermitian Transpose2 : matrix_library/Hermitian Transpose
  MATLAB Function : MATLAB Function  TreatAsAtomicUnit=on
  MATLAB Function1 : MATLAB Function  TreatAsAtomicUnit=on
  Matrix Multiply1 : Product  Multiplication=Matrix(*)
  Matrix Multiply2 : Product  Multiplication=Matrix(*)
  Mux1 : Mux  Inputs=3
  Mux2 : Mux  Inputs=3
  Reshape : Reshape  OutputDimensionality=Customize  OutputDimensions=[3,1]
  Scope : Scope
      settings: ActiveDisplayYMinimum=-1219.3822  ActiveDisplayYMaximum=10974.4399
  Stop Simulation : Stop  Commented=on
  Subtract : Sum  Inputs=+-
  Switch1 : Switch  Commented=on  Criteria=u2 > Threshold  SaturateOnIntegerOverflow=off  InputSameDT=off
  To Workspace : ToWorkspace  Commented=on  VariableName=H_OUT  SaveFormat=Timeseries  SampleTime=-1
  tag scope: a_xyz=global, axg=global, ayg=global, azg=global, height=global, vg_xyz=global, vxg=global, vyg=global, vzg=global
  wires:
  [ax1] -> Mux1/1
  [theta_eular] -> MATLAB Function/2(theta)
  MATLAB Function/1(R_bg) -> Hermitian Transpose1/1
  [psi_eular] -> MATLAB Function/3(psi)
  [ay1] -> Mux1/2
  Mux1/1 -> Matrix Multiply1/2
  [phi_eular] -> MATLAB Function/1(phi)
  Matrix Multiply1/1 -> [a_xyz], Demux1/1
  [az1] -> Mux1/3
  Demux1/3 -> [azg]
  Demux1/1 -> [axg]
  Demux1/2 -> [ayg]
  Hermitian Transpose1/1 -> Matrix Multiply1/1
  Switch1/1 -> Stop Simulation/1
  From/1 -> Switch1/2
  Constant1/1 -> Switch1/1
  Constant2/1 -> Switch1/3
  Demux2/2 -> [vyg]
  [u] -> Mux2/1
  Demux2/3 -> [vzg]
  [w] -> Mux2/3
  Mux2/1 -> Matrix Multiply2/2
  [phi_eular] -> MATLAB Function1/1(phi)
  Matrix Multiply2/1 -> Reshape/1, Demux2/1
  Hermitian Transpose2/1 -> Matrix Multiply2/1
  [v] -> Mux2/2
  [theta_eular] -> MATLAB Function1/2(theta)
  [psi_eular] -> MATLAB Function1/3(psi)
  Demux2/1 -> [vxg]
  MATLAB Function1/1(R_bg) -> Hermitian Transpose2/1
  [Z_positon] -> Subtract/2
  Constant/1 -> Subtract/1
  Subtract/1 -> [height]
  Reshape/1 -> [vg_xyz]

== system takeoff23b/6DOF-MODEL/动力学/rotation EQ ==
  L : Inport
  M : Inport  Port=2
  N : Inport  Port=3
  Constant : Constant  Value=I
  Demux : Demux  Outputs=3
  Display3 : Display
  Gain : Gain  Gain=inv(I)  Multiplication=Matrix(K*u) (u vector)
  Integrator : Integrator
  Integrator1 : Integrator
  Integrator2 : Integrator
  MATLAB Function1 : MATLAB Function  TreatAsAtomicUnit=on
  Mux : Mux  Inputs=3
  Mux1 : Mux  Inputs=3
  Product : Product  Inputs=3  Multiplication=Matrix(*)
  Reshape : Reshape  OutputDimensionality=Column vector (2-D)
  Reshape1 : Reshape
  Reshape2 : Reshape  OutputDimensionality=Column vector (2-D)
  Subsystem3 : Subsystem  Commented=on
  Sum : Sum  Inputs=|+-
  Sum1 : Sum  Inputs=|++
  p : Outport  VectorParamsAs1DForOutWhenUnconnected=off
  q : Outport  Port=2  VectorParamsAs1DForOutWhenUnconnected=off
  r : Outport  Port=3  VectorParamsAs1DForOutWhenUnconnected=off
  wires:
  Mux/1 -> Reshape/1, Display3/1
  Sum/1 -> Gain/1
  Demux/1 -> Integrator/1
  Demux/2 -> Integrator2/1
  Demux/3 -> Integrator1/1
  Gain/1 -> Reshape1/1
  Reshape1/1 -> Demux/1
  N/1 -> Mux/3
  L/1 -> Mux/1
  M/1 -> Mux/2
  Product/1 -> Sum/2
  MATLAB Function1/1(wB_X) -> Product/1
  Constant/1 -> Product/2
  Integrator/1 -> p/1, Mux1/1
  Integrator1/1 -> r/1, Mux1/3
  Integrator2/1 -> q/1, Mux1/2
  Reshape2/1 -> Product/3
  Mux1/1 -> Reshape2/1, MATLAB Function1/1(w)
  Reshape/1 -> Sum1/1
  [M_gear] -> Sum1/2
  Sum1/1 -> Sum/1

== system takeoff23b/6DOF-MODEL/动力学/姿态角 ==
  p : Inport
  q : Inport  Port=2
  r : Inport  Port=3
  Subsystem : Subsystem
  Subsystem1 : Subsystem
  Subsystem2 : Subsystem
  phi(eular) : Outport
  theta(eular) : Outport  Port=2
  psi(eular) : Outport  Port=3
  tag scope: phi_eular=global, psi_eular=global, theta_eular=global
  wires:
  q/1 -> Subsystem2/1(q), Subsystem1/1(q), Subsystem/2(q)
  Subsystem2/1(psi(euler)) -> [psi_eular], psi(eular)/1
  r/1 -> Subsystem2/2(r), Subsystem1/2(r), Subsystem/3(r)
  Subsystem/1(phi(euler)) -> Subsystem1/3(phi(euler)), Subsystem2/3(phi(euler)), phi(eular)/1, [phi_eular]
  Subsystem1/1(theta(euler)) -> Subsystem/4(theta(euler)), theta(eular)/1, [theta_eular], Subsystem2/4(theta(euler))
  p/1 -> Subsystem/1(p)

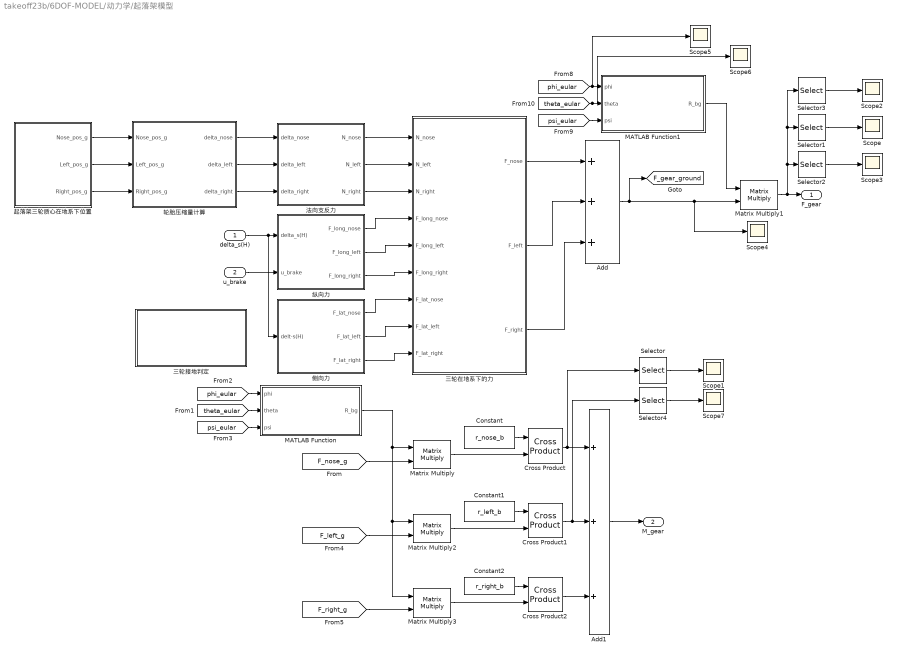
== system takeoff23b/6DOF-MODEL/动力学/起落架模型 ==
  delta_s(H) : Inport
  u_brake : Inport  Port=2
  Add : Sum  Inputs=+++
  Add1 : Sum  Inputs=+++
  Constant : Constant  Value=r_nose_b
  Constant1 : Constant  Value=r_left_b
  Constant2 : Constant  Value=r_right_b
  Cross Product : matrix_library/Cross Product
  Cross Product1 : matrix_library/Cross Product
  Cross Product2 : matrix_library/Cross Product
  MATLAB Function : MATLAB Function  TreatAsAtomicUnit=on
  MATLAB Function1 : MATLAB Function  TreatAsAtomicUnit=on
  Matrix Multiply{,1..3} (4 alike) : Product  Multiplication=Matrix(*)
  Scope{,1..7} (8 alike) : Scope
      Scope settings: ActiveDisplayYMinimum=-0.12099  ActiveDisplayYMaximum=0.34578  DataLoggingVariableName=ScopeData10
      Scope1 settings: ActiveDisplayYMinimum=-1  ActiveDisplayYMaximum=1  DataLoggingVariableName=ScopeData24
      Scope2 settings: ActiveDisplayYMinimum=-83.9341  ActiveDisplayYMaximum=93.9708
      Scope3 settings: ActiveDisplayYMinimum=-2.566918678712E+8  ActiveDisplayYMaximum=5.740525821668E+8  DataLoggingVariableName=ScopeData2
      Scope4 settings: ActiveDisplayYMinimum=-0.18022  ActiveDisplayYMaximum=0.17037  DataLoggingVariableName=ScopeData3
      Scope5 settings: ActiveDisplayYMinimum=1E-13  ActiveDisplayYMaximum=2.6E-13  DataLoggingVariableName=ScopeData4
      Scope6 settings: ActiveDisplayYMinimum=-1.962  ActiveDisplayYMaximum=1.9629  DataLoggingVariableName=ScopeData5
      Scope7 settings: ActiveDisplayYMinimum=-973.3061  ActiveDisplayYMaximum=108.1451  DataLoggingVariableName=ScopeData4
  Selector : Selector  InputPortWidth=3  IndexOptions=Index vector (dialog)  Indices=3  OutputSizes=1
  Selector1 : Selector  InputPortWidth=3  IndexOptions=Index vector (dialog)  Indices=2  OutputSizes=1
  Selector2 : Selector  InputPortWidth=3  IndexOptions=Index vector (dialog)  Indices=3  OutputSizes=1
  Selector3 : Selector  InputPortWidth=3  IndexOptions=Index vector (dialog)  Indices=1  OutputSizes=1
  Selector4 : Selector  InputPortWidth=3  IndexOptions=Index vector (dialog)  Indices=3  OutputSizes=1
  三轮在地系下的力 : Subsystem
  三轮接地判定 : Subsystem
  侧向力 : Subsystem
  法向支反力 : Subsystem
  纵向力 : Subsystem
  起落架三轮质心在地系下位置 : Subsystem
  轮胎压缩量计算 : Subsystem
  F_gear : Outport
  M_gear : Outport  Port=2
  tag scope: F_gear_ground=global
  wires:
  起落架三轮质心在地系下位置/1(Nose_pos_g) -> 轮胎压缩量计算/1(Nose_pos_g)
  起落架三轮质心在地系下位置/2(Left_pos_g) -> 轮胎压缩量计算/2(Left_pos_g)
  起落架三轮质心在地系下位置/3(Right_pos_g) -> 轮胎压缩量计算/3(Right_pos_g)
  轮胎压缩量计算/1(delta_nose) -> 法向支反力/1(delta_nose)
  轮胎压缩量计算/2(delta_left) -> 法向支反力/2(delta_left)
  轮胎压缩量计算/3(delta_right) -> 法向支反力/3(delta_right)
  delta_s(H)/1 -> 侧向力/1(delt-s(H)), 纵向力/1(delta_s(H))
  u_brake/1 -> 纵向力/2(u_brake)
  法向支反力/1(N_nose) -> 三轮在地系下的力/1(N_nose)
  法向支反力/2(N_left) -> 三轮在地系下的力/2(N_left)
  法向支反力/3(N_right) -> 三轮在地系下的力/3(N_right)
  纵向力/1(F_long_nose) -> 三轮在地系下的力/4(F_long_nose)
  纵向力/2(F_long_left) -> 三轮在地系下的力/5(F_long_left)
  纵向力/3(F_long_right) -> 三轮在地系下的力/6(F_long_right)
  侧向力/1(F_lat_nose) -> 三轮在地系下的力/7(F_lat_nose)
  侧向力/2(F_lat_left) -> 三轮在地系下的力/8(F_lat_left)
  侧向力/3(F_lat_right) -> 三轮在地系下的力/9(F_lat_right)
  三轮在地系下的力/1(F_nose) -> Add/1
  三轮在地系下的力/2(F_left) -> Add/2
  三轮在地系下的力/3(F_right) -> Add/3
  Add/1 -> Scope4/1, Matrix Multiply1/2, [F_gear_ground]
  MATLAB Function1/1(R_bg) -> Matrix Multiply1/1
  [phi_eular] -> MATLAB Function1/1(phi), Scope5/1
  Matrix Multiply1/1 -> Selector3/1, Selector1/1, Selector2/1, F_gear/1
  Constant/1 -> Cross Product/1
  Constant1/1 -> Cross Product1/1
  Constant2/1 -> Cross Product2/1
  Cross Product/1 -> Add1/1, Selector/1
  Cross Product1/1 -> Selector4/1, Add1/2
  Cross Product2/1 -> Add1/3
  Add1/1 -> M_gear/1
  [theta_eular] -> Scope6/1, MATLAB Function1/2(theta)
  [psi_eular] -> MATLAB Function1/3(psi)
  [theta_eular] -> MATLAB Function/2(theta)
  [phi_eular] -> MATLAB Function/1(phi)
  [psi_eular] -> MATLAB Function/3(psi)
  MATLAB Function/1(R_bg) -> Matrix Multiply3/1, Matrix Multiply2/1, Matrix Multiply/1
  [F_nose_g] -> Matrix Multiply/2
  [F_right_g] -> Matrix Multiply3/2
  [F_left_g] -> Matrix Multiply2/2
  Matrix Multiply2/1 -> Cross Product1/2
  Matrix Multiply3/1 -> Cross Product2/2
  Matrix Multiply/1 -> Cross Product/2
  Selector1/1 -> Scope/1
  Selector3/1 -> Scope2/1
  Selector2/1 -> Scope3/1
  Selector/1 -> Scope1/1
  Selector4/1 -> Scope7/1

== system takeoff23b/Flight Phase Manager/Data Pre-processing/Subsystem ==
  判断条件 : Inport
  Compare To Constant15 : simulink/Logic and Bit Operations/Compare To Constant  relop=>=  const=1  OutDataTypeStr=boolean
  Constant1 : Constant
  Integrator1 : Integrator  ExternalReset=level
  Logical Operator6 : Logic  Operator=NOT  AllPortsSameDT=off  OutDataTypeStr=boolean
  out : Outport
  wires:
  判断条件/1 -> Logical Operator6/1
  Compare To Constant15/1 -> out/1
  Integrator1/1 -> Compare To Constant15/1
  Logical Operator6/1 -> Integrator1/2
  Constant1/1 -> Integrator1/1

== system takeoff23b/Flight Phase Manager/Data Pre-processing/Subsystem1 ==
  判断条件 : Inport
  Compare To Constant15 : simulink/Logic and Bit Operations/Compare To Constant  relop=>=  const=1  OutDataTypeStr=boolean
  Constant1 : Constant
  Integrator1 : Integrator  ExternalReset=level
  Logical Operator6 : Logic  Operator=NOT  AllPortsSameDT=off  OutDataTypeStr=boolean
  out : Outport
  wires:
  判断条件/1 -> Logical Operator6/1
  Compare To Constant15/1 -> out/1
  Integrator1/1 -> Compare To Constant15/1
  Logical Operator6/1 -> Integrator1/2
  Constant1/1 -> Integrator1/1

== system takeoff23b/Flight Phase Manager/Data Pre-processing/Subsystem2 ==
  判断条件 : Inport
  Compare To Constant15 : simulink/Logic and Bit Operations/Compare To Constant  relop=>=  const=1  OutDataTypeStr=boolean
  Constant1 : Constant
  Integrator1 : Integrator  ExternalReset=level
  Logical Operator6 : Logic  Operator=NOT  AllPortsSameDT=off  OutDataTypeStr=boolean
  out : Outport
  wires:
  Constant1/1 -> Integrator1/1
  Logical Operator6/1 -> Integrator1/2
  Integrator1/1 -> Compare To Constant15/1
  Compare To Constant15/1 -> out/1
  判断条件/1 -> Logical Operator6/1

== system takeoff23b/Flight Phase Manager/Data Pre-processing/Subsystem3 ==
  判断条件 : Inport
  Compare To Constant15 : simulink/Logic and Bit Operations/Compare To Constant  relop=>=  const=1  OutDataTypeStr=boolean
  Constant1 : Constant
  Integrator1 : Integrator  ExternalReset=level
  Logical Operator6 : Logic  Operator=NOT  AllPortsSameDT=off  OutDataTypeStr=boolean
  out : Outport
  wires:
  Constant1/1 -> Integrator1/1
  Logical Operator6/1 -> Integrator1/2
  Integrator1/1 -> Compare To Constant15/1
  Compare To Constant15/1 -> out/1
  判断条件/1 -> Logical Operator6/1

== system takeoff23b/Flight Phase Manager/Data Pre-processing/Subsystem4 ==
  判断条件 : Inport
  Compare To Constant15 : simulink/Logic and Bit Operations/Compare To Constant  relop=>=  const=1  OutDataTypeStr=boolean
  Constant1 : Constant
  Integrator1 : Integrator  ExternalReset=level
  Logical Operator6 : Logic  Operator=NOT  AllPortsSameDT=off  OutDataTypeStr=boolean
  out : Outport
  wires:
  Constant1/1 -> Integrator1/1
  Logical Operator6/1 -> Integrator1/2
  Integrator1/1 -> Compare To Constant15/1
  Compare To Constant15/1 -> out/1
  判断条件/1 -> Logical Operator6/1

== system takeoff23b/Flight Phase Manager/Data Pre-processing/Subsystem5 ==
  判断条件 : Inport
  Compare To Constant15 : simulink/Logic and Bit Operations/Compare To Constant  relop=>=  const=1  OutDataTypeStr=boolean
  Constant1 : Constant
  Integrator1 : Integrator  ExternalReset=level
  Logical Operator6 : Logic  Operator=NOT  AllPortsSameDT=off  OutDataTypeStr=boolean
  out : Outport
  wires:
  判断条件/1 -> Logical Operator6/1
  Compare To Constant15/1 -> out/1
  Integrator1/1 -> Compare To Constant15/1
  Logical Operator6/1 -> Integrator1/2
  Constant1/1 -> Integrator1/1

== system takeoff23b/Flight Phase Manager/Data Pre-processing/Subsystem6 ==
  判断条件 : Inport
  Compare To Constant15 : simulink/Logic and Bit Operations/Compare To Constant  relop=>=  const=1  OutDataTypeStr=boolean
  Constant1 : Constant
  Integrator1 : Integrator  ExternalReset=level
  Logical Operator6 : Logic  Operator=NOT  AllPortsSameDT=off  OutDataTypeStr=boolean
  out : Outport
  wires:
  Constant1/1 -> Integrator1/1
  Logical Operator6/1 -> Integrator1/2
  Integrator1/1 -> Compare To Constant15/1
  Compare To Constant15/1 -> out/1
  判断条件/1 -> Logical Operator6/1

== system takeoff23b/Flight Phase Manager/Data Pre-processing/持续1秒 ==
  判断条件 : Inport
  Compare To Constant15 : simulink/Logic and Bit Operations/Compare To Constant  relop=>=  const=1  OutDataTypeStr=boolean
  Constant1 : Constant
  Integrator1 : Integrator  ExternalReset=level
  Logical Operator6 : Logic  Operator=NOT  AllPortsSameDT=off  OutDataTypeStr=boolean
  out : Outport
  wires:
  Constant1/1 -> Integrator1/1
  Logical Operator6/1 -> Integrator1/2
  Integrator1/1 -> Compare To Constant15/1
  Compare To Constant15/1 -> out/1
  判断条件/1 -> Logical Operator6/1

== system takeoff23b/Flight Phase Manager/Data Pre-processing/持续1秒1 ==
  判断条件 : Inport
  Compare To Constant15 : simulink/Logic and Bit Operations/Compare To Constant  relop=>=  const=1  OutDataTypeStr=boolean
  Constant1 : Constant
  Integrator1 : Integrator  ExternalReset=level
  Logical Operator6 : Logic  Operator=NOT  AllPortsSameDT=off  OutDataTypeStr=boolean
  out : Outport
  wires:
  判断条件/1 -> Logical Operator6/1
  Compare To Constant15/1 -> out/1
  Integrator1/1 -> Compare To Constant15/1
  Logical Operator6/1 -> Integrator1/2
  Constant1/1 -> Integrator1/1

== system takeoff23b/Flight Phase Manager/Data Pre-processing/持续1秒2 ==
  判断条件 : Inport
  Compare To Constant15 : simulink/Logic and Bit Operations/Compare To Constant  relop=>=  const=1  OutDataTypeStr=boolean
  Constant1 : Constant
  Integrator1 : Integrator  ExternalReset=level
  Logical Operator6 : Logic  Operator=NOT  AllPortsSameDT=off  OutDataTypeStr=boolean
  out : Outport
  wires:
  判断条件/1 -> Logical Operator6/1
  Compare To Constant15/1 -> out/1
  Integrator1/1 -> Compare To Constant15/1
  Logical Operator6/1 -> Integrator1/2
  Constant1/1 -> Integrator1/1

== system takeoff23b/Flight Phase Manager/Data Pre-processing/持续1秒3 ==
  判断条件 : Inport
  Compare To Constant15 : simulink/Logic and Bit Operations/Compare To Constant  relop=>=  const=1  OutDataTypeStr=boolean
  Constant1 : Constant
  Integrator1 : Integrator  ExternalReset=level
  Logical Operator6 : Logic  Operator=NOT  AllPortsSameDT=off  OutDataTypeStr=boolean
  out : Outport
  wires:
  判断条件/1 -> Logical Operator6/1
  Compare To Constant15/1 -> out/1
  Integrator1/1 -> Compare To Constant15/1
  Logical Operator6/1 -> Integrator1/2
  Constant1/1 -> Integrator1/1
